simulink model "HypersonicSimulation"  (R2021b)
settings: Solver=ode4  StartTime=0.0  StopTime=1800  FixedStep=0.1  RelTol=1e-3
undefined symbols (not defined in the file or in its folder): a, AlphaTab, alt, C_D, C_Da, C_L, C_La, CTvq, Ispvq, press, rho, temp
libraries: aerolibconvert2 x6, slpidlib x3, simulink x2
settings Model: PacingRate=5  Creator=Owner  LastModifiedBy=Owner

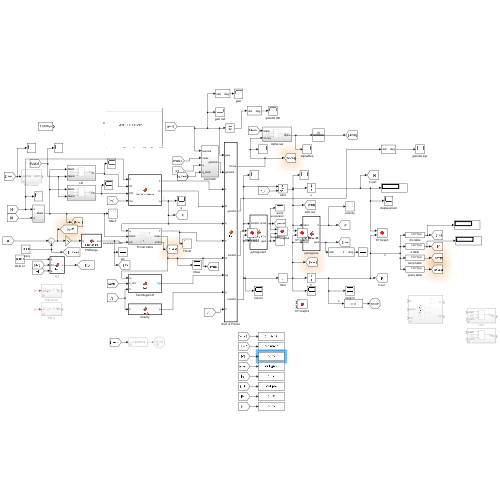
[thumbnail: Simulink's stored preview of the top-level diagram]
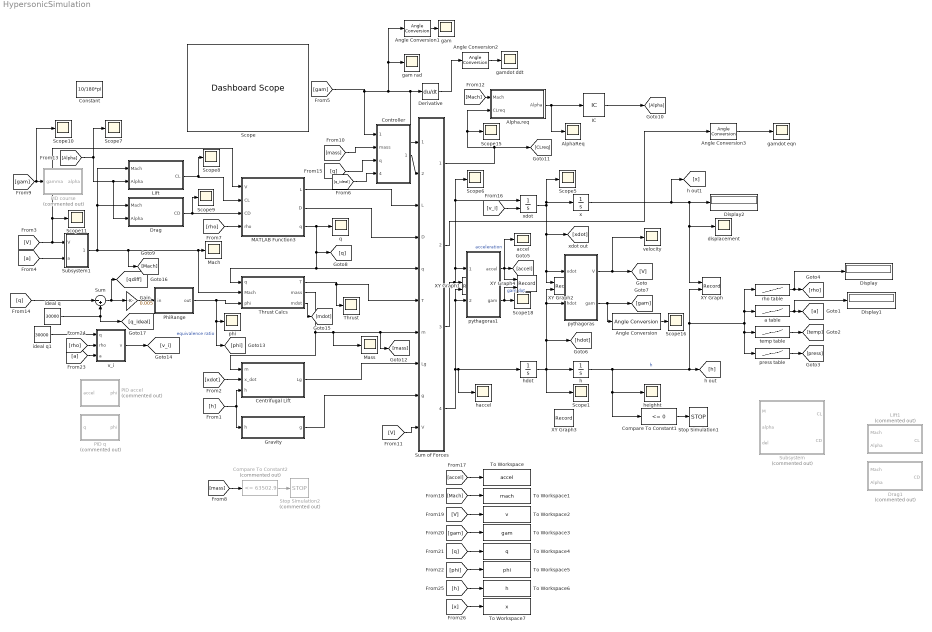
== system HypersonicSimulation ==
  Alpha,req : Subsystem
  AlphaReq : Scope
  Angle Conversion{,1..3} (4 alike) : aerolibconvert2/Angle Conversion  IU=rad  OU=deg
  Centrifugal Lift : MATLAB Function  TreatAsAtomicUnit=on
  Compare To Constant1 : simulink/Logic and Bit Operations/Compare To Constant  relop=<=  const=0  OutDataTypeStr=boolean
  Compare To Constant2 : simulink/Logic and Bit Operations/Compare To Constant  Commented=on  relop=<=  const=63502.9  OutDataTypeStr=boolean
  Constant : Constant  Value=10/180*pi
  Controller : Subsystem
  Derivative : Derivative
  Display : Display
  Display1 : Display
  Display2 : Display
  Drag : Subsystem
  Drag1 : Subsystem  Commented=on
  Gain : Gain  Gain=0.005
  Gravity : MATLAB Function  TreatAsAtomicUnit=on
  IC : InitialCondition
  Lift : Subsystem
  Lift1 : Subsystem  Commented=on
  MATLAB Function3 : MATLAB Function  TreatAsAtomicUnit=on
  Mach : Scope
  Mass : Scope
  PID accel : Subsystem  Commented=on
  PID course : Subsystem  Commented=on
  PID q : Subsystem  Commented=on
  PhiRange : MATLAB Function  TreatAsAtomicUnit=on
  Scope : DashboardScope  Ymin=0  Ymax=100  Markers=on
  Scope{1,5..11,15..16,18} (11 alike) : Scope
  Stop Simulation1 : Stop
  Stop Simulation2 : Stop  Commented=on
  Subsystem : Subsystem  Commented=on
  Subsystem1 : Subsystem
  Sum : Sum  Inputs=|-+
  Sum of Forces : MATLAB Function  TreatAsAtomicUnit=on
  Thrust : Scope
  Thrust Calcs : Subsystem
  To Workspace : ToWorkspace  VariableName=accel  SaveFormat=Timeseries  SampleTime=-1
  To Workspace1 : ToWorkspace  VariableName=mach  SampleTime=-1
  To Workspace2 : ToWorkspace  VariableName=v  SaveFormat=Timeseries  SampleTime=-1
  To Workspace3 : ToWorkspace  VariableName=gam  SaveFormat=Timeseries  SampleTime=-1
  To Workspace4 : ToWorkspace  VariableName=q  SampleTime=-1
  To Workspace5 : ToWorkspace  VariableName=phi  SaveFormat=Timeseries  SampleTime=-1
  To Workspace6 : ToWorkspace  VariableName=h  SampleTime=-1
  To Workspace7 : ToWorkspace  VariableName=x  SampleTime=-1
  XY Graph : Record  FileSettingsInternal="{\"entries\":[{\"content\":{\"excelSettings\":{\"content\":{},\"type\":\"Streamout.ExcelSettings\"}},\"type\":\"Streamout.FileSettingStorage\",\"uuid\":\"743886f9-634a-4fd6-8e1c-5824b6ef6ded\"}],\"packageUris\":[\"http://schema.mathworks.com/mf0/streamout_blocks/R2020a\"],\"version\":\"1.0\"}"  Layout=[1 1]  SignalsInternal="{\"entries\":[{\"content\":{\"signals\":[{\"content\":{\"blockPath\":[\"sim30kto13k/XY Graph\"],\"channel\":[],\"dimensions\":[1],\"domain\":\"sim30kto13k/XY Graph\",\"lineColor\":\"#ff6929\",\"plots\":[1],\"port\":1,\"sid\":[\"\"],\"signalID\":5323,\"signalName\":\"x\"},\"type\":\"RecordBlkView.Signal\",\"uuid\":\"c77f4e7b-694d-493f-9721-9f567deb40eb\"},{\"content\":{\"blockPath\":[\"sim30kto13k/XY Graph\"],\"channel\":[],\"dimensions\":[1],\"domain\":\"sim30kto13k/XY Graph\",\"lineColor\":\"#b746ff\",\"plots\":[1],\"port\":2,\"sid\":[\"\"],\"signalID\":5327,\"signalName\":\"h\"},\"type\":\"RecordBlkView.Signal\",\"uuid\":\"dce025af-7d4a-412c-b2a2-44bf9c8e5d17\"}]},\"type\":\"RecordBlkView.InputSignals\",\"uuid\":\"d7a24cfb-9764-4178-9fc3-ef918fa0fab2\"}],\"packageUris\":[\"http://schema.mathworks.com/mf0/streamout_blocks/R2020a\"],\"version\":\"1.0\"}"  VisualizationBindings="{\"xyplotplugin\":{\"info\":[{\"series\":[{\"bindingParametersList\":[{\"parameter\":\"X-Axis\",\"signalID\":5323,\"signalName\":\"x\"},{\"parameter\":\"Y-Axis\",\"signalID\":5327,\"signalName\":\"h\"}],\"seriesID\":64119}],\"subplotID\":1}]}}"  CompatibilityTag=XY
  XY Graph1 : Record  FileSettingsInternal="{\"entries\":[{\"content\":{\"excelSettings\":{\"content\":{},\"type\":\"Streamout.ExcelSettings\"}},\"type\":\"Streamout.FileSettingStorage\",\"uuid\":\"3e083810-543a-4c6b-919b-6308d8e7a27f\"}],\"packageUris\":[\"http://schema.mathworks.com/mf0/streamout_blocks/R2020a\"],\"version\":\"1.0\"}"  Layout=[1 1]  SignalsInternal="{\"entries\":[{\"content\":{\"signals\":[{\"content\":{\"blockPath\":[\"sim30kto13k/XY Graph1\"],\"channel\":[],\"dimensions\":[1],\"domain\":\"sim30kto13k/XY Graph1\",\"lineColor\":\"#a2142f\",\"plots\":[1],\"port\":1,\"sid\":[\"\"],\"signalID\":5331,\"signalName\":\"Sum of Forces:3\"},\"type\":\"RecordBlkView.Signal\",\"uuid\":\"c626b1ac-6459-4cda-9e18-20cc58a3938c\"},{\"content\":{\"blockPath\":[\"sim30kto13k/XY Graph1\"],\"channel\":[],\"dimensions\":[1],\"domain\":\"sim30kto13k/XY Graph1\",\"lineColor\":\"#139fff\",\"plots\":[1],\"port\":2,\"sid\":[\"\"],\"signalID\":5335,\"signalName\":\"Sum of Forces:4\"},\"type\":\"RecordBlkView.Signal\",\"uuid\":\"86d2c567-db74-4f06-8f82-bc1383f67a7c\"}]},\"type\":\"RecordBlkView.InputSignals\",\"uuid\":\"ef5d6253-86ea-4037-ad09-09d4994d043e\"}],\"packageUris\":[\"http://schema.mathworks.com/mf0/streamout_blocks/R2020a\"],\"version\":\"1.0\"}"  VisualizationBindings="{\"xyplotplugin\":{\"info\":[{\"series\":[{\"bindingParametersList\":[{\"parameter\":\"X-Axis\",\"signalID\":5331,\"signalName\":\"Sum of Forces:3\"},{\"parameter\":\"Y-Axis\",\"signalID\":5335,\"signalName\":\"Sum of Forces:4\"}],\"seriesID\":62508}],\"subplotID\":1}]}}"  CompatibilityTag=XY
  XY Graph2 : Record  FileSettingsInternal="{\"entries\":[{\"content\":{\"excelSettings\":{\"content\":{},\"type\":\"Streamout.ExcelSettings\"}},\"type\":\"Streamout.FileSettingStorage\",\"uuid\":\"763cf81b-296e-4a93-a510-dc087bb74c78\"}],\"packageUris\":[\"http://schema.mathworks.com/mf0/streamout_blocks/R2020a\"],\"version\":\"1.0\"}"  Layout=[1 1]  SignalsInternal="{\"entries\":[{\"content\":{\"signals\":[{\"content\":{\"blockPath\":[\"sim30kto13k/XY Graph2\"],\"channel\":[],\"dimensions\":[1],\"domain\":\"sim30kto13k/XY Graph2\",\"lineColor\":\"#0072bd\",\"plots\":[],\"port\":1,\"sid\":[\"\"],\"signalID\":5339,\"signalName\":\"xdot\"},\"type\":\"RecordBlkView.Signal\",\"uuid\":\"99682e9f-e405-46dc-9ec8-4b822dbef361\"},{\"content\":{\"blockPath\":[\"sim30kto13k/XY Graph2\"],\"channel\":[],\"dimensions\":[1],\"domain\":\"sim30kto13k/XY Graph2\",\"lineColor\":\"#d95319\",\"plots\":[],\"port\":2,\"sid\":[\"\"],\"signalID\":5343,\"signalName\":\"hdot\"},\"type\":\"RecordBlkView.Signal\",\"uuid\":\"d32e12f7-a9fd-4650-a8c4-381cb3a36308\"}]},\"type\":\"RecordBlkView.InputSignals\",\"uuid\":\"08cfc7f1-db32-493b-885b-5ac8281889cc\"}],\"packageUris\":[\"http://schema.mathworks.com/mf0/streamout_blocks/R2020a\"],\"version\":\"1.0\"}"  VisualizationBindings="{\"xyplotplugin\":{\"info\":[{\"series\":[],\"subplotID\":1}]}}"  CompatibilityTag=XY
  XY Graph3 : Record  FileSettingsInternal="{\"entries\":[{\"content\":{\"excelSettings\":{\"content\":{},\"type\":\"Streamout.ExcelSettings\"}},\"type\":\"Streamout.FileSettingStorage\",\"uuid\":\"476b5e19-3549-4328-a773-167e1908eb4a\"}],\"packageUris\":[\"http://schema.mathworks.com/mf0/streamout_blocks/R2020a\"],\"version\":\"1.0\"}"  Layout=[1 1]  SignalsInternal="{\"entries\":[{\"content\":{\"signals\":[{\"content\":{\"blockPath\":[\"sim30kto13k/XY Graph3\"],\"channel\":[],\"dimensions\":[1],\"domain\":\"sim30kto13k/XY Graph3\",\"lineColor\":\"#77ac30\",\"plots\":[],\"port\":1,\"sid\":[\"\"],\"signalID\":5355},\"type\":\"RecordBlkView.Signal\",\"uuid\":\"995cfb20-1940-4be5-acc0-e0eddb20fa1b\"},{\"content\":{\"blockPath\":[\"sim30kto13k/XY Graph3\"],\"channel\":[],\"dimensions\":[1],\"domain\":\"sim30kto13k/XY Graph3\",\"lineColor\":\"#4dbeee\",\"plots\":[],\"port\":2,\"sid\":[\"\"],\"signalID\":5359},\"type\":\"RecordBlkView.Signal\",\"uuid\":\"c53bb78e-f436-41ca-8783-4882cf9ca451\"}]},\"type\":\"RecordBlkView.InputSignals\",\"uuid\":\"afaf51e7-7c33-462e-9feb-564cf246fc44\"}],\"packageUris\":[\"http://schema.mathworks.com/mf0/streamout_blocks/R2020a\"],\"version\":\"1.0\"}"  VisualizationBindings="{\"xyplotplugin\":{\"info\":[{\"series\":[],\"subplotID\":1}]}}"  CompatibilityTag=XY
  XY Graph4 : Record  FileSettingsInternal="{\"entries\":[{\"content\":{\"excelSettings\":{\"content\":{},\"type\":\"Streamout.ExcelSettings\"}},\"type\":\"Streamout.FileSettingStorage\",\"uuid\":\"fc0ba5e1-7b5a-4160-91f5-03585b6db69d\"}],\"packageUris\":[\"http://schema.mathworks.com/mf0/streamout_blocks/R2020a\"],\"version\":\"1.0\"}"  Layout=[1 1]  SignalsInternal="{\"entries\":[{\"content\":{\"signals\":[{\"content\":{\"blockPath\":[\"sim30kto13k/XY Graph4\"],\"channel\":[],\"dimensions\":[1],\"domain\":\"sim30kto13k/XY Graph4\",\"lineColor\":\"#edb120\",\"plots\":[],\"port\":1,\"sid\":[\"\"],\"signalID\":5347,\"signalName\":\"acceleration\"},\"type\":\"RecordBlkView.Signal\",\"uuid\":\"ef5a9895-190d-4fb1-a3fb-11bc8bc4a9b4\"},{\"content\":{\"blockPath\":[\"sim30kto13k/XY Graph4\"],\"channel\":[],\"dimensions\":[1],\"domain\":\"sim30kto13k/XY Graph4\",\"lineColor\":\"#7e2f8e\",\"plots\":[],\"port\":2,\"sid\":[\"\"],\"signalID\":5351,\"signalName\":\"gam dot\"},\"type\":\"RecordBlkView.Signal\",\"uuid\":\"fbe869c5-c47c-450a-8e89-40410ab16dbc\"}]},\"type\":\"RecordBlkView.InputSignals\",\"uuid\":\"7f4b2f5c-749a-452b-beac-8543dcdb1dc6\"}],\"packageUris\":[\"http://schema.mathworks.com/mf0/streamout_blocks/R2020a\"],\"version\":\"1.0\"}"  VisualizationBindings="{\"xyplotplugin\":{\"info\":[{\"series\":[],\"subplotID\":1}]}}"  CompatibilityTag=XY
  a table : Lookup_n-D  NumberOfTableDimensions=1  BreakpointsForDimension1=alt  Table=a  InternalRulePriority=Speed  RndMeth=Simplest  InputSameDT=on
  accel : Scope
  displacement : Scope
  gam : Scope
  gam rad : Scope
  gamdot ddt : Scope
  gamdot eqn : Scope
  h : Integrator  InitialCondition=25000
  haccel : Scope
  hdot : Integrator
  heighht : Scope
  ideal q : Constant  Value=30000
  ideal q1 : Constant  Value=30000
  phi : Scope
  press table : Lookup_n-D  NumberOfTableDimensions=1  BreakpointsForDimension1=alt  Table=press  InternalRulePriority=Speed  RndMeth=Simplest  InputSameDT=on
  pythagoras : MATLAB Function  TreatAsAtomicUnit=on
  pythagoras1 : MATLAB Function  TreatAsAtomicUnit=on
  q : Scope
  rho table : Lookup_n-D  NumberOfTableDimensions=1  BreakpointsForDimension1=alt  Table=rho  InternalRulePriority=Speed  RndMeth=Simplest  InputSameDT=on
  temp table : Lookup_n-D  NumberOfTableDimensions=1  BreakpointsForDimension1=alt  Table=temp  InternalRulePriority=Speed  RndMeth=Simplest  InputSameDT=on
  v_i : MATLAB Function  TreatAsAtomicUnit=on
  velocity : Scope
  x : Integrator
  xdot : Integrator  InitialConditionSource=external  InitialCondition=1700
  wires:
  Thrust Calcs/1(T) -> Thrust/1, Sum of Forces/6(T)
  Centrifugal Lift/1(Lg) -> Sum of Forces/8(Lg)
  Sum of Forces/3(xdotdot) -> Scope6/1, xdot/1, pythagoras1/1(xdotdot), XY Graph1/1
  xdot/1 -> Scope5/1, x/1, XY Graph2/1, pythagoras/1(xdot), [xdot]
  Sum of Forces/4(hdotdot) -> haccel/1, hdot/1, pythagoras1/2(hdotdot), XY Graph1/2
  hdot/1 -> Scope1/1, XY Graph2/2, pythagoras/2(hdot), [hdot], h/1
  [h] -> Gravity/1(h), Centrifugal Lift/3(h)
  Gravity/1(g) -> Sum of Forces/9(g)
  MATLAB Function3/2(D) -> Sum of Forces/4(D)
  MATLAB Function3/1(L) -> Sum of Forces/3(L)
  pythagoras/1(V) -> velocity/1, [V]
  x/1 -> Display2/1, XY Graph/1, displacement/1, [x]
  [xdot] -> Centrifugal Lift/2(x_dot)
  Compare To Constant1/1 -> Stop Simulation1/1
  h/1 -> [h], XY Graph/2, press table/1, temp table/1, rho table/1, a table/1, heighht/1, Compare To Constant1/1  "h"
  pythagoras1/1(accel) -> XY Graph4/1, [accel], accel/1  "acceleration"
  pythagoras1/2(gam) -> XY Graph4/2, Scope18/1  "gam dot"
  Angle Conversion/1 -> Scope16/1
  [V] -> Scope11/1, MATLAB Function3/1(V), Subsystem1/1(V)
  [a] -> Subsystem1/2(a)
  rho table/1 -> Display/1, [rho]
  press table/1 -> [press]
  temp table/1 -> [temp]
  a table/1 -> Display1/1, [a]
  Subsystem1/1(Mach) -> Drag/1(Mach), Lift/1(Mach), [Mach], Mach/1, Thrust Calcs/2(Mach)
  MATLAB Function3/3(q) -> Sum of Forces/5(q), Thrust Calcs/1(q), [q], q/1
  [rho] -> MATLAB Function3/4(rho)
  ? -> PID accel/1(accel)
  pythagoras/2(gam) -> [gam], Angle Conversion/1
  Drag/1(CD) -> Scope9/1, MATLAB Function3/3(CD)
  Lift/1(CL) -> MATLAB Function3/2(CL), Scope8/1
  [Alpha] -> Drag/2(Alpha), Lift/2(Alpha), Scope7/1
  [gam] -> Scope10/1, PID course/1(gamma)
  [gam] -> gam rad/1, Angle Conversion1/1, Sum of Forces/1(gam), Derivative/1, Controller/1(Gamma)
  ? -> PID q/1(q)
  [V] -> Sum of Forces/10(V)
  [Mach] -> Alpha,req/1(Mach)
  Controller/1(gamdoti) -> Sum of Forces/2(gamdoti)
  Gain/1 -> PhiRange/1(in)
  Thrust Calcs/2(mass) -> Mass/1, Sum of Forces/7(m), [mass], Centrifugal Lift/1(m)
  Derivative/1 -> Angle Conversion2/1
  [mass] -> Controller/2(mass)
  Angle Conversion1/1 -> gam/1
  Angle Conversion2/1 -> gamdot ddt/1
  Sum of Forces/2(gamdot) -> Angle Conversion3/1
  Angle Conversion3/1 -> gamdot eqn/1
  [v_i] -> xdot/2
  [accel] -> To Workspace/1
  [Mach] -> To Workspace1/1
  [V] -> To Workspace2/1
  [gam] -> To Workspace3/1
  [q] -> To Workspace4/1
  [phi] -> To Workspace5/1
  [a] -> v_i/3(a)
  [rho] -> v_i/2(rho)
  v_i/1(v) -> [v_i]
  Thrust Calcs/3(mdot) -> [mdot]
  ideal q/1 -> [q_ideal], Sum/2
  Sum/1 -> [qdiff], Gain/1
  PhiRange/1(out) -> Thrust Calcs/3(phi), [phi], phi/1  "equivalence ratio"
  [q] -> Sum/1
  Sum of Forces/1(CLreq) -> Scope15/1, Alpha,req/2(CLreq), [CLreq]
  [q] -> Controller/3(q)
  Alpha,req/1(Alpha) -> IC/1, AlphaReq/1
  IC/1 -> [Alpha]
  [q_ideal] -> Controller/4(q_ideal)
  Compare To Constant2/1 -> Stop Simulation2/1
  [mass] -> Compare To Constant2/1
  ideal q1/1 -> v_i/1(q)
  [h] -> To Workspace6/1
  [x] -> To Workspace7/1

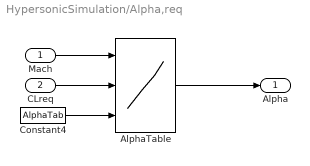
== system HypersonicSimulation/Alpha,req ==
  Mach : Inport
  CLreq : Inport  Port=2
  AlphaTable : Lookup_n-D  BreakpointsForDimension1=[0.3 0.7 0.9 1.5 2.5 4 6 10 15 20 24]  BreakpointsForDimension2=[-0.5:0.01:0.5]  TableSource=Input port  InternalRulePriority=Speed  RndMeth=Simplest  InputSameDT=on
      settings: InputPortMap=u0,u1,p221
  Constant4 : Constant  Value=AlphaTab  VectorParams1D=off
  Alpha : Outport
  wires:
  Constant4/1 -> AlphaTable/3
  CLreq/1 -> AlphaTable/2
  Mach/1 -> AlphaTable/1
  AlphaTable/1 -> Alpha/1

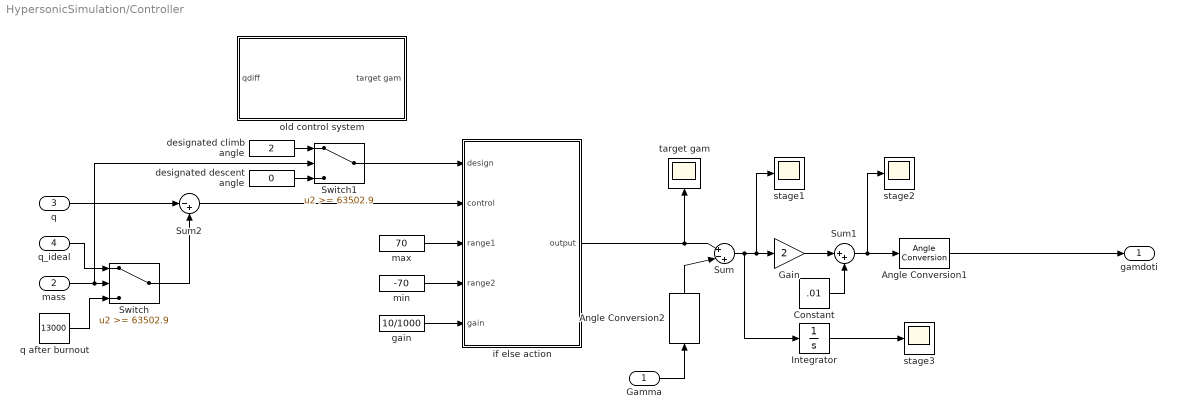
== system HypersonicSimulation/Controller ==
  Gamma : Inport
  mass : Inport  Port=2
  q : Inport  Port=3
  q_ideal : Inport  Port=4
  Angle Conversion1 : aerolibconvert2/Angle Conversion  IU=deg  OU=rad
  Angle Conversion2 : aerolibconvert2/Angle Conversion  IU=rad  OU=deg
  Constant : Constant  Value=.01
  Gain : Gain  Gain=2
  Integrator : Integrator
  Sum : Sum  Inputs=|+-+
  Sum1 : Sum  Inputs=|++
  Sum2 : Sum  Inputs=|-+
  Switch : Switch  Threshold=63502.9
  Switch1 : Switch  Threshold=63502.9
  designated climb angle : Constant  Value=2
  designated descent angle : Constant  Value=0
  gain : Constant  Value=10/1000
  if else action : MATLAB Function  TreatAsAtomicUnit=on
  max : Constant  Value=70
  min : Constant  Value=-70
  old control system : Subsystem
  q after burnout : Constant  Value=13000
  stage1 : Scope
  stage2 : Scope
  stage3 : Scope
  target gam : Scope
  gamdoti : Outport
  wires:
  Gamma/1 -> Angle Conversion2/1
  Sum/1 -> Integrator/1, stage1/1, Gain/1
  Gain/1 -> Sum1/1
  Sum1/1 -> stage2/1, Angle Conversion1/1
  Constant/1 -> Sum1/2
  Angle Conversion2/1 -> Sum/2
  Integrator/1 -> stage3/1
  if else action/1(output) -> target gam/1, Sum/1
  Angle Conversion1/1 -> gamdoti/1
  q_ideal/1 -> Switch/1
  q after burnout/1 -> Switch/3
  Switch/1 -> Sum2/2
  mass/1 -> Switch1/2, Switch/2
  q/1 -> Sum2/1
  Sum2/1 -> if else action/2(control)
  Switch1/1 -> if else action/1(design)
  max/1 -> if else action/3(range1)
  gain/1 -> if else action/5(gain)
  min/1 -> if else action/4(range2)
  designated descent angle/1 -> Switch1/3
  designated climb angle/1 -> Switch1/1

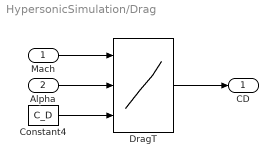
== system HypersonicSimulation/Drag ==
  Mach : Inport
  Alpha : Inport  Port=2
  Constant4 : Constant  Value=C_D  VectorParams1D=off
  DragT : Lookup_n-D  BreakpointsForDimension1=[0.3 0.7 0.9 1.5 2.5 4 6 10 15 20 24]  BreakpointsForDimension2=[-15 -12 -10 -8 -6 -4 -2 -1 0 1 2 4 6 8 10 12 15]  TableSource=Input port  InternalRulePriority=Speed  RndMeth=Simplest  InputSameDT=on
      settings: InputPortMap=u0,u1,p221
  CD : Outport
  wires:
  Constant4/1 -> DragT/3
  Alpha/1 -> DragT/2
  DragT/1 -> CD/1
  Mach/1 -> DragT/1

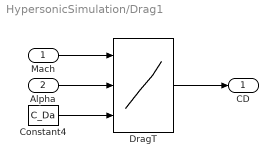
== system HypersonicSimulation/Drag1 ==
  Mach : Inport
  Alpha : Inport  Port=2
  Constant4 : Constant  Value=C_Da  VectorParams1D=off
  DragT : Lookup_n-D  BreakpointsForDimension1=[0.3 0.7 0.9 1.5 2.5 4 6 10 15 20 24]  BreakpointsForDimension2=|  TableSource=Input port  InternalRulePriority=Speed  RndMeth=Simplest  InputSameDT=on
      | [-1
      | 0
      | 1
      | 2
      | 4
      | 6
      | 8
      | 10
      | 12]
      settings: InputPortMap=u0,u1,p221
  CD : Outport
  wires:
  Constant4/1 -> DragT/3
  Alpha/1 -> DragT/2
  DragT/1 -> CD/1
  Mach/1 -> DragT/1

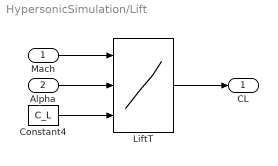
== system HypersonicSimulation/Lift ==
  Mach : Inport
  Alpha : Inport  Port=2
  Constant4 : Constant  Value=C_L  VectorParams1D=off
  LiftT : Lookup_n-D  BreakpointsForDimension1=[0.3 0.7 0.9 1.5 2.5 4 6 10 15 20 24]  BreakpointsForDimension2=[-15 -12 -10 -8 -6 -4 -2 -1 0 1 2 4 6 8 10 12 15]  TableSource=Input port  InternalRulePriority=Speed  RndMeth=Simplest  InputSameDT=on
      settings: InputPortMap=u0,u1,p221
  CL : Outport
  wires:
  Mach/1 -> LiftT/1
  LiftT/1 -> CL/1
  Alpha/1 -> LiftT/2
  Constant4/1 -> LiftT/3

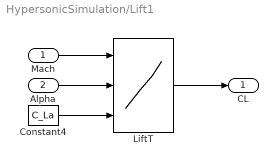
== system HypersonicSimulation/Lift1 ==
  Mach : Inport
  Alpha : Inport  Port=2
  Constant4 : Constant  Value=C_La  VectorParams1D=off
  LiftT : Lookup_n-D  BreakpointsForDimension1=[0.3 0.7 0.9 1.5 2.5 4 6 10 15 20 24]  BreakpointsForDimension2=|  TableSource=Input port  InternalRulePriority=Speed  RndMeth=Simplest  InputSameDT=on
      | [-1
      | 0
      | 1
      | 2
      | 4
      | 6
      | 8
      | 10
      | 12]
      settings: InputPortMap=u0,u1,p221
  CL : Outport
  wires:
  Mach/1 -> LiftT/1
  LiftT/1 -> CL/1
  Alpha/1 -> LiftT/2
  Constant4/1 -> LiftT/3

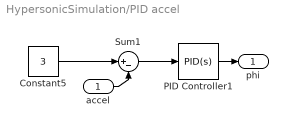
== system HypersonicSimulation/PID accel ==
  accel : Inport
  Constant5 : Constant  Value=3
  PID Controller1 : slpidlib/PID Controller  Controller=PID  Form=Parallel  TimeDomain=Continuous-time  UseExternalTs=off  SampleTime=-1  IntegratorMethod=Forward Euler  FilterMethod=Forward Euler  ControllerParametersSource=internal  P=0  I=2.70577796557585  D=0  UseFilter=on  N=100  TunerSelectOption=Transfer Function Based (PID Tuner App)  InitialConditionSource=internal  InitialConditionForIntegrator=0  InitialConditionForFilter=0  DifferentiatorICPrevScaledInput=0  ExternalReset=none  TrackingMode=off  Kt=1  LimitOutput=off  SatLimitsSource=internal  UpperSaturationLimit=inf  LowerSaturationLimit=-inf  LinearizeAsGain=on  AntiWindupMode=none  Kb=1  POutMin=[]  POutMax=[]  IOutMin=[]  IOutMax=[]  DOutMin=[]  DOutMax=[]  NOutMin=[]  NOutMax=[]  SumOutMin=[]  SumOutMax=[]  SaturationOutMin=[]  SaturationOutMax=[]  PParamMin=[]  PParamMax=[]  IParamMin=[]  IParamMax=[]  DParamMin=[]  DParamMax=[]  NParamMin=[]  NParamMax=[]  KbParamMin=[]  KbParamMax=[]  KtParamMin=[]  KtParamMax=[]  KbOutMin=[]  KbOutMax=[]  KtOutMin=[]  KtOutMax=[]  IntegratorOutMin=[]  IntegratorOutMax=[]  FilterOutMin=[]  FilterOutMax=[]  SumI1OutMin=[]  SumI1OutMax=[]  SumI2OutMin=[]  SumI2OutMax=[]  SumI3OutMin=[]  SumI3OutMax=[]  SumI4OutMin=[]  SumI4OutMax=[]  SumDOutMin=[]  SumDOutMax=[]  DifferentiatorOutMin=[]  DifferentiatorOutMax=[]  FilterDiffOutCoefMin=[]  FilterDiffOutCoefMax=[]  ReciprocalOutMin=[]  ReciprocalOutMax=[]  SumDenOutMin=[]  SumDenOutMax=[]  SumNumOutMin=[]  SumNumOutMax=[]  DivideOutMin=[]  DivideOutMax=[]  UdiffTsProdOutMin=[]  UdiffTsProdOutMax=[]  NTsProdOutMin=[]  NTsProdOutMax=[]  UintegralTsProdOutMin=[]  UintegralTsProdOutMax=[]  UngainTsProdOutMin=[]  UngainTsProdOutMax=[]  IntegratorContinuousStateAttributes=''  IntegratorStateMustResolveToSignalObject=off  IntegratorRTWStateStorageClass=Auto  FilterContinuousStateAttributes=''  FilterStateMustResolveToSignalObject=off  FilterRTWStateStorageClass=Auto  ParallelPVariant=InternalParameters  IdealPVariant=Disabled  IVariant=InternalParameters  DVariant=InternalParameters  IntegratorVariant=Continuous  SatVariant=Disabled  AWVariant=Passthrough  PCopyVariant=Disabled  TRVariant=Disabled  FdbkBlocksVariant=Forward  IdealPFdbkVariant=Disabled  SatFdbkVariant=Disabled  DerivativeFilterVariant=ContFilter  NVariant=InternalParameters  NCopyVariant=Disabled  FilterICVariant=InternalICsFilter  IntegratorICVariant=InternalICs  ExternalResetVariant=Disabled  TRSumVariant=Passthrough  SumFdbkVariant=Disabled  SumVariant=Sum_PID  TsampFilterVariant=InternalTs  TsampNgainVariant=Passthrough  TsampIntegralVariant=Passthrough  ExternalSaturationOutDataTypeStr=Inherit: Same as second input
  Sum1 : Sum  Inputs=|+-
  phi : Outport
  wires:
  accel/1 -> Sum1/2
  PID Controller1/1 -> phi/1
  Constant5/1 -> Sum1/1
  Sum1/1 -> PID Controller1/1

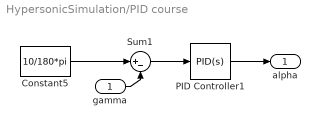
== system HypersonicSimulation/PID course ==
  gamma : Inport
  Constant5 : Constant  Value=10/180*pi
  PID Controller1 : slpidlib/PID Controller  Controller=PID  Form=Parallel  TimeDomain=Continuous-time  UseExternalTs=off  SampleTime=-1  IntegratorMethod=Forward Euler  FilterMethod=Forward Euler  ControllerParametersSource=internal  P=3  I=1  D=90.9663911465854  UseFilter=on  N=50  TunerSelectOption=Transfer Function Based (PID Tuner App)  InitialConditionSource=internal  InitialConditionForIntegrator=0  InitialConditionForFilter=0  DifferentiatorICPrevScaledInput=0  ExternalReset=none  TrackingMode=off  Kt=1  LimitOutput=off  SatLimitsSource=internal  UpperSaturationLimit=inf  LowerSaturationLimit=-inf  LinearizeAsGain=on  AntiWindupMode=none  Kb=1  POutMin=[]  POutMax=[]  IOutMin=[]  IOutMax=[]  DOutMin=[]  DOutMax=[]  NOutMin=[]  NOutMax=[]  SumOutMin=[]  SumOutMax=[]  SaturationOutMin=[]  SaturationOutMax=[]  PParamMin=[]  PParamMax=[]  IParamMin=[]  IParamMax=[]  DParamMin=[]  DParamMax=[]  NParamMin=[]  NParamMax=[]  KbParamMin=[]  KbParamMax=[]  KtParamMin=[]  KtParamMax=[]  KbOutMin=[]  KbOutMax=[]  KtOutMin=[]  KtOutMax=[]  IntegratorOutMin=[]  IntegratorOutMax=[]  FilterOutMin=[]  FilterOutMax=[]  SumI1OutMin=[]  SumI1OutMax=[]  SumI2OutMin=[]  SumI2OutMax=[]  SumI3OutMin=[]  SumI3OutMax=[]  SumI4OutMin=[]  SumI4OutMax=[]  SumDOutMin=[]  SumDOutMax=[]  DifferentiatorOutMin=[]  DifferentiatorOutMax=[]  FilterDiffOutCoefMin=[]  FilterDiffOutCoefMax=[]  ReciprocalOutMin=[]  ReciprocalOutMax=[]  SumDenOutMin=[]  SumDenOutMax=[]  SumNumOutMin=[]  SumNumOutMax=[]  DivideOutMin=[]  DivideOutMax=[]  UdiffTsProdOutMin=[]  UdiffTsProdOutMax=[]  NTsProdOutMin=[]  NTsProdOutMax=[]  UintegralTsProdOutMin=[]  UintegralTsProdOutMax=[]  UngainTsProdOutMin=[]  UngainTsProdOutMax=[]  IntegratorContinuousStateAttributes=''  IntegratorStateMustResolveToSignalObject=off  IntegratorRTWStateStorageClass=Auto  FilterContinuousStateAttributes=''  FilterStateMustResolveToSignalObject=off  FilterRTWStateStorageClass=Auto  ParallelPVariant=InternalParameters  IdealPVariant=Disabled  IVariant=InternalParameters  DVariant=InternalParameters  IntegratorVariant=Continuous  SatVariant=Disabled  AWVariant=Passthrough  PCopyVariant=Disabled  TRVariant=Disabled  FdbkBlocksVariant=Forward  IdealPFdbkVariant=Disabled  SatFdbkVariant=Disabled  DerivativeFilterVariant=ContFilter  NVariant=InternalParameters  NCopyVariant=Disabled  FilterICVariant=InternalICsFilter  IntegratorICVariant=InternalICs  ExternalResetVariant=Disabled  TRSumVariant=Passthrough  SumFdbkVariant=Disabled  SumVariant=Sum_PID  TsampFilterVariant=InternalTs  TsampNgainVariant=Passthrough  TsampIntegralVariant=Passthrough  ExternalSaturationOutDataTypeStr=Inherit: Same as second input
  Sum1 : Sum  Inputs=|+-
  alpha : Outport
  wires:
  Sum1/1 -> PID Controller1/1
  Constant5/1 -> Sum1/1
  PID Controller1/1 -> alpha/1
  gamma/1 -> Sum1/2

== system HypersonicSimulation/PID q ==
  q : Inport
  Constant5 : Constant  Value=40000
  PID Controller1 : slpidlib/PID Controller  Controller=PID  Form=Parallel  TimeDomain=Continuous-time  UseExternalTs=off  SampleTime=-1  IntegratorMethod=Forward Euler  FilterMethod=Forward Euler  ControllerParametersSource=internal  P=0.00981293241423901  I=0.00143403581608144  D=-0.00131790791672402  UseFilter=on  N=1.10912614685618  TunerSelectOption=Transfer Function Based (PID Tuner App)  InitialConditionSource=internal  InitialConditionForIntegrator=0  InitialConditionForFilter=0  DifferentiatorICPrevScaledInput=0  ExternalReset=none  TrackingMode=off  Kt=1  LimitOutput=off  SatLimitsSource=internal  UpperSaturationLimit=inf  LowerSaturationLimit=-inf  LinearizeAsGain=on  AntiWindupMode=none  Kb=1  POutMin=[]  POutMax=[]  IOutMin=[]  IOutMax=[]  DOutMin=[]  DOutMax=[]  NOutMin=[]  NOutMax=[]  SumOutMin=[]  SumOutMax=[]  SaturationOutMin=[]  SaturationOutMax=[]  PParamMin=[]  PParamMax=[]  IParamMin=[]  IParamMax=[]  DParamMin=[]  DParamMax=[]  NParamMin=[]  NParamMax=[]  KbParamMin=[]  KbParamMax=[]  KtParamMin=[]  KtParamMax=[]  KbOutMin=[]  KbOutMax=[]  KtOutMin=[]  KtOutMax=[]  IntegratorOutMin=[]  IntegratorOutMax=[]  FilterOutMin=[]  FilterOutMax=[]  SumI1OutMin=[]  SumI1OutMax=[]  SumI2OutMin=[]  SumI2OutMax=[]  SumI3OutMin=[]  SumI3OutMax=[]  SumI4OutMin=[]  SumI4OutMax=[]  SumDOutMin=[]  SumDOutMax=[]  DifferentiatorOutMin=[]  DifferentiatorOutMax=[]  FilterDiffOutCoefMin=[]  FilterDiffOutCoefMax=[]  ReciprocalOutMin=[]  ReciprocalOutMax=[]  SumDenOutMin=[]  SumDenOutMax=[]  SumNumOutMin=[]  SumNumOutMax=[]  DivideOutMin=[]  DivideOutMax=[]  UdiffTsProdOutMin=[]  UdiffTsProdOutMax=[]  NTsProdOutMin=[]  NTsProdOutMax=[]  UintegralTsProdOutMin=[]  UintegralTsProdOutMax=[]  UngainTsProdOutMin=[]  UngainTsProdOutMax=[]  IntegratorContinuousStateAttributes=''  IntegratorStateMustResolveToSignalObject=off  IntegratorRTWStateStorageClass=Auto  FilterContinuousStateAttributes=''  FilterStateMustResolveToSignalObject=off  FilterRTWStateStorageClass=Auto  ParallelPVariant=InternalParameters  IdealPVariant=Disabled  IVariant=InternalParameters  DVariant=InternalParameters  IntegratorVariant=Continuous  SatVariant=Disabled  AWVariant=Passthrough  PCopyVariant=Disabled  TRVariant=Disabled  FdbkBlocksVariant=Forward  IdealPFdbkVariant=Disabled  SatFdbkVariant=Disabled  DerivativeFilterVariant=ContFilter  NVariant=InternalParameters  NCopyVariant=Disabled  FilterICVariant=InternalICsFilter  IntegratorICVariant=InternalICs  ExternalResetVariant=Disabled  TRSumVariant=Passthrough  SumFdbkVariant=Disabled  SumVariant=Sum_PID  TsampFilterVariant=InternalTs  TsampNgainVariant=Passthrough  TsampIntegralVariant=Passthrough  ExternalSaturationOutDataTypeStr=Inherit: Same as second input
  Sum1 : Sum  Inputs=|+-
  phi : Outport
  wires:
  Sum1/1 -> PID Controller1/1
  Constant5/1 -> Sum1/1
  PID Controller1/1 -> phi/1
  q/1 -> Sum1/2

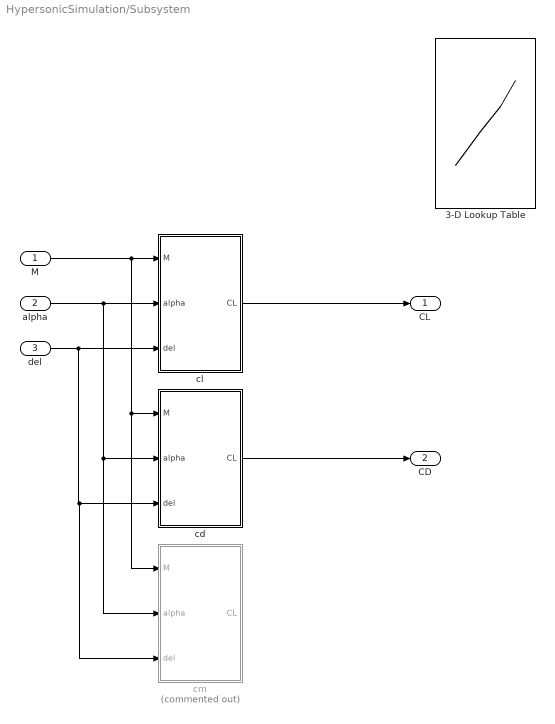
== system HypersonicSimulation/Subsystem ==
  M : Inport
  alpha : Inport  Port=2
  del : Inport  Port=3
  3-D Lookup Table : Lookup_n-D  BreakpointsForDimension1Source=Input port  BreakpointsForDimension2Source=Input port  BreakpointsForDimension3=[5, 7]  TableSource=Input port  Table=reshape(repmat([4 5 6;16 19 20;10 18 23],1,2),[3,3,2])  InternalRulePriority=Speed  RndMeth=Simplest  InputSameDT=on
      settings: InputPortMap=u0,u1,p221,p5,p7
  cd : MATLAB Function  TreatAsAtomicUnit=on
  cl : MATLAB Function  TreatAsAtomicUnit=on
  cm : MATLAB Function  Commented=on  TreatAsAtomicUnit=on
  CL : Outport
  CD : Outport  Port=2
  wires:
  M/1 -> cm/1(M), cd/1(M), cl/1(M)
  alpha/1 -> cl/2(alpha), cd/2(alpha), cm/2(alpha)
  del/1 -> cm/3(del), cd/3(del), cl/3(del)
  cl/1(CL) -> CL/1
  cd/1(CL) -> CD/1

== system HypersonicSimulation/Subsystem1 ==
  V : Inport
  a : Inport  Port=2
  Product1 : Product  Inputs=*/  InputSameDT=on  SaturateOnIntegerOverflow=on  OutDataTypeStr=Inherit: Same as first input
  Mach : Outport  Unit=1  VectorParamsAs1DForOutWhenUnconnected=off
  wires:
  Product1/1 -> Mach/1
  V/1 -> Product1/1
  a/1 -> Product1/2

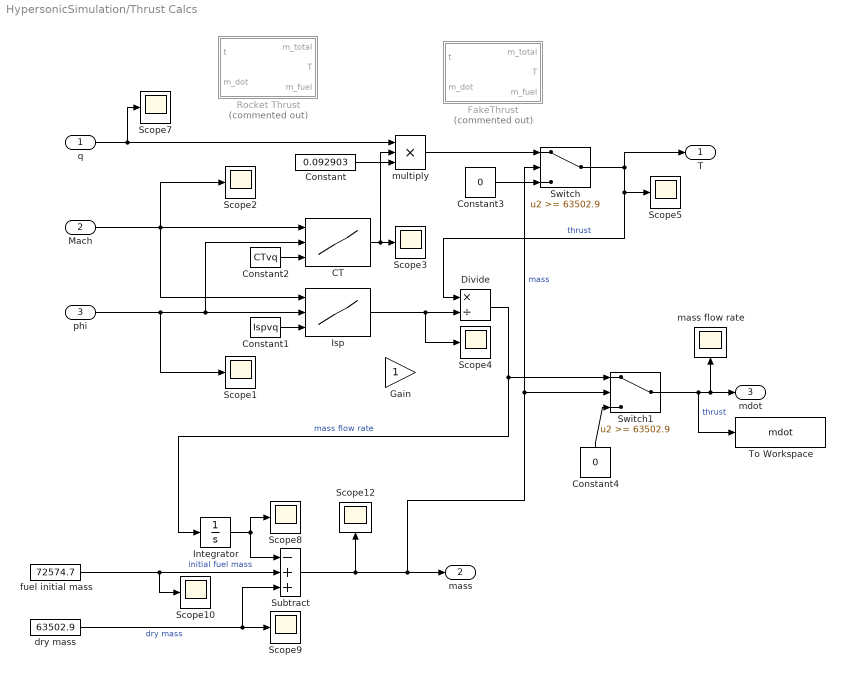
== system HypersonicSimulation/Thrust Calcs ==
  q : Inport
  Mach : Inport  Port=2
  phi : Inport  Port=3
  CT : Lookup_n-D  BreakpointsForDimension1=[0:0.1:25]  BreakpointsForDimension2=[0:0.1:10]  TableSource=Input port  InternalRulePriority=Speed  RndMeth=Simplest  InputSameDT=on
      settings: InputPortMap=u0,u1,p221
  Constant : Constant  Value=0.092903
  Constant1 : Constant  Value=Ispvq  VectorParams1D=off
  Constant2 : Constant  Value=CTvq  VectorParams1D=off
  Constant3 : Constant  Value=0
  Constant4 : Constant  Value=0
  Divide : Product  Inputs=*/
  FakeThrust : MATLAB Function  Commented=on  TreatAsAtomicUnit=on
  Gain : Gain
  Integrator : Integrator  InitialCondition=100
  Isp : Lookup_n-D  BreakpointsForDimension1=[0:0.1:25]  BreakpointsForDimension2=[0:0.1:10]  TableSource=Input port  InternalRulePriority=Speed  RndMeth=Simplest  InputSameDT=on
      settings: InputPortMap=u0,u1,p221
  Rocket Thrust : MATLAB Function  Commented=on  TreatAsAtomicUnit=on
  Scope{1..5,7..10,12} (10 alike) : Scope
  Subtract : Sum  Inputs=-++
  Switch : Switch  Threshold=63502.9
  Switch1 : Switch  Threshold=63502.9
  To Workspace : ToWorkspace  VariableName=mdot  SampleTime=-1
      settings: Save2DSignal=2-D array (concatenate along first dimension)
  dry mass : Constant  Value=63502.9
  fuel initial mass : Constant  Value=72574.7
  mass flow rate : Scope
  multiply : Product  Inputs=***
  T : Outport
  mass : Outport  Port=2
  mdot : Outport  Port=3
  wires:
  q/1 -> Scope7/1, multiply/1
  Isp/1 -> Scope4/1, Divide/2
  phi/1 -> CT/2, Isp/2, Scope1/1
  Constant2/1 -> CT/3
  CT/1 -> multiply/2, Scope3/1
  Constant1/1 -> Isp/3
  Mach/1 -> CT/1, Scope2/1, Isp/1
  Constant/1 -> multiply/3
  Integrator/1 -> Subtract/1, Scope8/1
  dry mass/1 -> Scope9/1, Subtract/3  "dry mass"
  Subtract/1 -> mass/1, Switch1/2, Switch/2, Scope12/1  "mass"
  fuel initial mass/1 -> Scope10/1, Subtract/2  "initial fuel mass"
  Divide/1 -> Switch1/1, Integrator/1  "mass flow rate"
  multiply/1 -> Switch/1
  Switch/1 -> T/1, Scope5/1, Divide/1  "thrust"
  Constant3/1 -> Switch/3
  Constant4/1 -> Switch1/3
  Switch1/1 -> mass flow rate/1, mdot/1, To Workspace/1  "thrust"

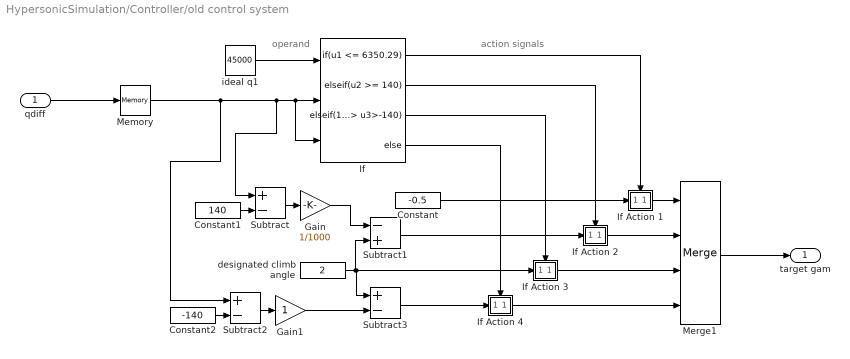
== system HypersonicSimulation/Controller/old control system ==
  note: action signals
  note: operand
  qdiff : Inport
  Constant : Constant  Value=-0.5
  Constant1 : Constant  Value=140
  Constant2 : Constant  Value=-140
  Gain : Gain  Gain=1/1000
  Gain1 : Gain
  If : If  NumInputs=3  IfExpression=u1 <= 6350.29  ElseIfExpressions=u2 >= 140, 140> u3>-140
  If Action 1 : Subsystem  TreatAsAtomicUnit=on
  If Action 2 : Subsystem  TreatAsAtomicUnit=on
  If Action 3 : Subsystem  TreatAsAtomicUnit=on
  If Action 4 : Subsystem  TreatAsAtomicUnit=on
  Memory : Memory
  Merge1 : Merge  Inputs=4
  Subtract : Sum  Inputs=+-
  Subtract1 : Sum  Inputs=-+
  Subtract2 : Sum  Inputs=+-
  Subtract3 : Sum  Inputs=+-
  designated climb angle : Constant  Value=2
  ideal q1 : Constant  Value=45000
  target gam : Outport
  wires:
  Gain/1 -> Subtract1/1
  If Action 3/1(Out1) -> Merge1/3
  Memory/1 -> Subtract2/1, Subtract/1, If/2, If/3
  If Action 1/1(Out1) -> Merge1/1
  If Action 2/1(Out1) -> Merge1/2
  If Action 4/1(Out1) -> Merge1/4
  qdiff/1 -> Memory/1
  If/2 -> If Action 2/Action
  If/1 -> If Action 1/Action
  Merge1/1 -> target gam/1
  Constant/1 -> If Action 1/1(Action 1)
  designated climb angle/1 -> Subtract1/2, Subtract3/1, If Action 3/1(Action 3)
  Gain1/1 -> Subtract3/2
  If/3 -> If Action 3/Action
  If/4 -> If Action 4/Action
  ideal q1/1 -> If/1
  Subtract/1 -> Gain/1
  Constant2/1 -> Subtract2/2
  Subtract1/1 -> If Action 2/1(Action 2)
  Subtract2/1 -> Gain1/1
  Subtract3/1 -> If Action 4/1(Action 4)
  Constant1/1 -> Subtract/2

== system HypersonicSimulation/Controller/old control system/If Action 1 ==
  Action 1 : Inport
  Action Port : ActionPort  ActionPortLabel=if(u1 <= 6350.29)
  Out1 : Outport  VectorParamsAs1DForOutWhenUnconnected=off
  wires:
  Action 1/1 -> Out1/1

== system HypersonicSimulation/Controller/old control system/If Action 2 ==
  Action 2 : Inport
  Action Port : ActionPort  ActionPortLabel=elseif(u2 >= 140)
  Out1 : Outport  VectorParamsAs1DForOutWhenUnconnected=off
  wires:
  Action 2/1 -> Out1/1

== system HypersonicSimulation/Controller/old control system/If Action 3 ==
  Action 3 : Inport
  Action Port : ActionPort  ActionPortLabel=elseif( 140> u3>-140)
  Out1 : Outport  VectorParamsAs1DForOutWhenUnconnected=off
  wires:
  Action 3/1 -> Out1/1

== system HypersonicSimulation/Controller/old control system/If Action 4 ==
  Action 4 : Inport
  Action Port : ActionPort  ActionPortLabel=else
  Out1 : Outport  VectorParamsAs1DForOutWhenUnconnected=off
  wires:
  Action 4/1 -> Out1/1

== matlab function HypersonicSimulation/PhiRange ==
  data: in input; out output
function out = PhiRange(in)
if in <=0;
    out = 0;
elseif in >=5;
    out = 5;
else
    out = in;
end

== matlab function HypersonicSimulation/Subsystem/cd ==
  data: M input; CL output; alpha input; del input
function CL = fcn(M, alpha, del)
CLa = -5.2491e-004+alpha.* 1.5746e-002+(alpha.*M).*6.0213e-003 ...
    -3.4437e-004*alpha.^2+((alpha.*M).^2) * 1.4471E-04- ...
    5.1952E-05* alpha.^ 3+3.4771E-05*alpha.^ 4+2.7717E-03* M ^ 4 ...
    -2.3034E-06*alpha.^ 5
CLdel =-5.119E-04+1.000E-03*alpha-1.406E-04*(alpha*del)+1.313E-03*(alpha*M)...
    -8.584E-04* (M* del)+8.879E-05* (alpha* M)* del-1.604E-04* M^ 2-3.477E-04* alpha^2 ...
    -9.788E-05* (alpha* M)^ 2-1.703E-06* (M* del)^ 2+2.532E-05* alpha^ 3-3.727E-05* del^ 3 ...
    +1.781E-07* del^ 2+7.912E-07* ((alpha* M)* del)^ 2+2.465E-08* (alpha* del)^ 2 ...
    -9.788E-05* (alpha* M)^ 2-5.942E-09*((alpha* M)* del)^ 3 ...
    -7.377E-08* alpha^ 4+2.672E-08* del4-1.610E-11* ((alpha* M)* del)^ 4 ...
    -3.273E-08* alpha^ 5+7.624E-08* del^5+1.388E-13*((alpha* M)* del)^ 5;

CL = CLa+CLdel*2;

== matlab function HypersonicSimulation/Subsystem/cm ==
  data: M input; CL output; alpha input; del input
function CL = fcn(M, alpha, del)
CLa = -5.2491e-004+alpha.* 1.5746e-002+(alpha.*M).*6.0213e-003 ...
    -3.4437e-004*alpha.^2+((alpha.*M).^2) * 1.4471E-04- ...
    5.1952E-05* alpha.^ 3+3.4771E-05*alpha.^ 4+2.7717E-03* M ^ 4 ...
    -2.3034E-06*alpha.^ 5
CLdel =-5.119E-04+1.000E-03*alpha-1.406E-04*(alpha*del)+1.313E-03*(alpha*M)...
    -8.584E-04* (M* del)+8.879E-05* (alpha* M)* del-1.604E-04* M^ 2-3.477E-04* alpha^2 ...
    -9.788E-05* (alpha* M)^ 2-1.703E-06* (M* del)^ 2+2.532E-05* alpha^ 3-3.727E-05* del^ 3 ...
    +1.781E-07* del^ 2+7.912E-07* ((alpha* M)* del)^ 2+2.465E-08* (alpha* del)^ 2 ...
    -9.788E-05* (alpha* M)^ 2-5.942E-09*((alpha* M)* del)^ 3 ...
    -7.377E-08* alpha^ 4+2.672E-08* del4-1.610E-11* ((alpha* M)* del)^ 4 ...
    -3.273E-08* alpha^ 5+7.624E-08* del^5+1.388E-13*((alpha* M)* del)^ 5;

CL = CLa+CLdel*2;

== matlab function HypersonicSimulation/Thrust Calcs/FakeThrust ==
  data: m_total output; t input; T output; m_dot input; m_fuel output
function [m_total,T,m_fuel] = thrust(t,m_dot)
T=1000;
m_dry = 400;
m_fuel= 400-t*m_dot;
if m_fuel <= 0;
    T=0;
    m_fuel=0;
end
m_total=m_dry+m_fuel;

== matlab function HypersonicSimulation/Thrust Calcs/Rocket Thrust ==
  data: m_total output; t input; T output; m_dot input; m_fuel output
function [m_total,T,m_fuel] = thrust(t,m_dot)
T=1000;
m_dry = 400;
m_fuel= 400-t*m_dot;
if m_fuel <= 0;
    T=0;
    m_fuel=0;
end
m_total=m_dry+m_fuel;

== matlab function HypersonicSimulation/MATLAB Function3 ==
  data: V input; CL input; CD input; L output; D output; q output; rho input
function [L,D,q] = Aerodynamics(V,CL,CD,rho)
A=334.72;
q=0.5*rho*V^2;
L=q*CL*A;
D=q*CD*A;

== matlab function HypersonicSimulation/pythagoras1 ==
  data: accel output; xdotdot input; hdotdot input; gam output
function [accel, gam]= pythagoras(xdotdot,hdotdot)
accel=sqrt(xdotdot^2+hdotdot^2);
gam = atan(hdotdot/xdotdot);

== matlab function HypersonicSimulation/Sum of Forces ==
  data: gam input; gamdoti input; CLreq output; gamdot output; L input; D input; q input; T input; m input; xdotdot output; Lg input; g input; hdotdot output; V input
function [CLreq,gamdot,xdotdot,hdotdot]= Fx(gam,gamdoti, L,D,q,T,m,Lg,g,V)

xdotdot = 1/m*(T*cos(gam)-D*cos(gam)-L*sin(gam)-Lg*cos(gam)*sin(gam));
hdotdot = 1/m*(Lg*cos(gam)^2+L*cos(gam)-m*g+T*sin(gam)-D*sin(gam));

gamdot = 1/(m*V)*(Lg*cos(gam)+L-m*g*cos(gam));

A=334.72;
CLreq = 1/q/A*(m*g*cos(gam) - Lg*cos(gam)+ gamdoti*m*V/30);

== matlab function HypersonicSimulation/v_i ==
  data: q input; v output; rho input; a input
function v = fcn(q,rho,a)
v = sqrt(2*q/rho);

== matlab function HypersonicSimulation/Centrifugal Lift ==
  data: Lg output; m input; x_dot input; h input
function Lg  = Lg(m,x_dot,h)
Re=6378e3;
Lg=m*x_dot^2/(Re+h);

== matlab function HypersonicSimulation/Controller/if else action ==
  data: design input; output output; control input; range1 input; range2 input; gain input
function output = fcn(design, control, range1, range2, gain)
if control>range1
    output = design - (control-range1)*gain;
elseif range1>=control>=range2
    output = design;
else
    output = design - (control-range2)*gain;
end

== matlab function HypersonicSimulation/Gravity ==
  data: g output; h input
function g = gravity(h)
% g0 = 9.80665
Re = 6378e3;
g0 = 9.7803;
g=g0*(Re/(Re+h))^2;

== matlab function HypersonicSimulation/pythagoras ==
  data: V output; xdot input; hdot input; gam output
function [V, gam] = pythagoras(xdot,hdot)
V=sqrt(xdot^2+hdot^2);
gam = atan(hdot/xdot);
% if xdot<0;
%     gam = pi+gam;
% end

== matlab function HypersonicSimulation/Subsystem/cl ==
  data: M input; CL output; alpha input; del input
function CL = fcn(M, alpha, del)
CLa = -5.2491e-004+alpha.* 1.5746e-002+(alpha.*M).*6.0213e-003 ...
    -3.4437e-004*alpha.^2+((alpha.*M).^2) * 1.4471E-04- ...
    5.1952E-05* alpha.^ 3+3.4771E-05*alpha.^ 4+2.7717E-03* M ^ 4 ...
    -2.3034E-06*alpha.^ 5
CLdel =-5.119E-04+1.000E-03*alpha-1.406E-04*(alpha*del)+1.313E-03*(alpha*M)...
    -8.584E-04* (M* del)+8.879E-05* (alpha* M)* del-1.604E-04* M^ 2-3.477E-04* alpha^2 ...
    -9.788E-05* (alpha* M)^ 2-1.703E-06* (M* del)^ 2+2.532E-05* alpha^ 3-3.727E-05* del^ 3 ...
    +1.781E-07* del^ 2+7.912E-07* ((alpha* M)* del)^ 2+2.465E-08* (alpha* del)^ 2 ...
    -9.788E-05* (alpha* M)^ 2-5.942E-09*((alpha* M)* del)^ 3 ...
    -7.377E-08* alpha^ 4+2.672E-08* del^4-1.610E-11* ((alpha* M)* del)^ 4 ...
    -3.273E-08* alpha^ 5+7.624E-08* del^5+1.388E-13*((alpha* M)* del)^ 5;

CL = CLa+CLdel*2;
